simulink model "ddc_bpm_476_066"  (Simulink 7.8)
settings: Solver=ode45  StartTime=0.0  StopTime=2e-3  RelTol=1e-3
undefined symbols (not defined in the file): decim_factor_poly_35, dt_sim, frev_476, Fs_adc, n_ch, n_ovs, R_fofb, R_sec, R_sec_cfir, R_sec_pfir, xlipgetpartsetting
libraries: xbsIndex_r4 x1436, simulink x7
(part 12 of 12)

== system ddc_bpm_476_066/TBT_amp/TBT_amp1/TBT_poly_decim/TDDM_TBT/TDDM_tbt_poly_i ==
  din : Inport
  ch_in : Inport  Port=2
  Constant : xbsIndex_r4/Constant  const=1  gui_display_data_type=Fixed-point  arith_type=Unsigned  n_bits=1  bin_pt=0  preci_type=Single  exp_width=8  frac_width=24  explicit_period=off  period=1  equ=P=C  opselect=C  inp2=PCIN>>17  opr=+  inp1=P  carry=CIN  dbl_ovrd=off  block_type=constant
  Constant1 : xbsIndex_r4/Constant  const=0  gui_display_data_type=Fixed-point  arith_type=Unsigned  n_bits=1  bin_pt=0  preci_type=Single  exp_width=8  frac_width=24  explicit_period=off  period=1  equ=P=C  opselect=C  inp2=PCIN>>17  opr=+  inp1=P  carry=CIN  dbl_ovrd=off  block_type=constant
  Delay : xbsIndex_r4/Delay  rst=off  infoeditControl=Selection of Reset will increase slice count due to use of real FFs and instead of SRLs  en=off  latency=3  dbl_ovrd=off  reg_retiming=off  block_type=delay
  Down Sample1 : xbsIndex_r4/Down Sample  sample_ratio=n_ch/n_ovs  sample_phase="Last Value of Frame  (most efficient)"  en=off  latency=1  dbl_ovrd=off  block_type=dsamp
  Down Sample2 : xbsIndex_r4/Down Sample  sample_ratio=n_ch/n_ovs  sample_phase="Last Value of Frame  (most efficient)"  en=off  latency=1  dbl_ovrd=off  block_type=dsamp
  Register : xbsIndex_r4/Register  init=0  rst=off  en=on  dbl_ovrd=off  block_type=register
  Register1 : xbsIndex_r4/Register  init=0  rst=off  en=on  dbl_ovrd=off  block_type=register
  Relational : xbsIndex_r4/Relational  mode=a=b  en=off  latency=1  dbl_ovrd=off  block_type=relational
  Relational1 : xbsIndex_r4/Relational  mode=a=b  en=off  latency=1  dbl_ovrd=off  block_type=relational
  dout_ch0 : Outport
  dout_ch1 : Outport  Port=2
  ch_out : Outport  Port=3
  wires:
  Constant/1 -> Relational/2
  Constant1/1 -> Relational1/2
  Relational/1 -> Register/2
  Relational1/1 -> Register1/2
  din/1 -> Register/1, Register1/1
  Register/1 -> Down Sample2/1
  ch_in/1 -> Relational/1, Relational1/1, Delay/1
  Register1/1 -> Down Sample1/1
  Down Sample2/1 -> dout_ch0/1
  Delay/1 -> ch_out/1
  Down Sample1/1 -> dout_ch1/1

== system ddc_bpm_476_066/TBT_amp/TBT_amp1/TBT_poly_decim/TDDM_TBT/TDDM_tbt_poly_q ==
  din : Inport
  ch_in : Inport  Port=2
  Constant : xbsIndex_r4/Constant  const=1  gui_display_data_type=Fixed-point  arith_type=Unsigned  n_bits=1  bin_pt=0  preci_type=Single  exp_width=8  frac_width=24  explicit_period=off  period=1  equ=P=C  opselect=C  inp2=PCIN>>17  opr=+  inp1=P  carry=CIN  dbl_ovrd=off  block_type=constant
  Constant1 : xbsIndex_r4/Constant  const=0  gui_display_data_type=Fixed-point  arith_type=Unsigned  n_bits=1  bin_pt=0  preci_type=Single  exp_width=8  frac_width=24  explicit_period=off  period=1  equ=P=C  opselect=C  inp2=PCIN>>17  opr=+  inp1=P  carry=CIN  dbl_ovrd=off  block_type=constant
  Delay : xbsIndex_r4/Delay  rst=off  infoeditControl=Selection of Reset will increase slice count due to use of real FFs and instead of SRLs  en=off  latency=3  dbl_ovrd=off  reg_retiming=off  block_type=delay
  Down Sample1 : xbsIndex_r4/Down Sample  sample_ratio=n_ch/n_ovs  sample_phase="Last Value of Frame  (most efficient)"  en=off  latency=1  dbl_ovrd=off  block_type=dsamp
  Down Sample2 : xbsIndex_r4/Down Sample  sample_ratio=n_ch/n_ovs  sample_phase="Last Value of Frame  (most efficient)"  en=off  latency=1  dbl_ovrd=off  block_type=dsamp
  Register : xbsIndex_r4/Register  init=0  rst=off  en=on  dbl_ovrd=off  block_type=register
  Register1 : xbsIndex_r4/Register  init=0  rst=off  en=on  dbl_ovrd=off  block_type=register
  Relational : xbsIndex_r4/Relational  mode=a=b  en=off  latency=1  dbl_ovrd=off  block_type=relational
  Relational1 : xbsIndex_r4/Relational  mode=a=b  en=off  latency=1  dbl_ovrd=off  block_type=relational
  dout_ch0 : Outport
  dout_ch1 : Outport  Port=2
  ch_out : Outport  Port=3
  wires:
  Constant/1 -> Relational/2
  Constant1/1 -> Relational1/2
  Relational/1 -> Register/2
  Relational1/1 -> Register1/2
  din/1 -> Register/1, Register1/1
  Register/1 -> Down Sample2/1
  ch_in/1 -> Relational/1, Relational1/1, Delay/1
  Register1/1 -> Down Sample1/1
  Down Sample2/1 -> dout_ch0/1
  Delay/1 -> ch_out/1
  Down Sample1/1 -> dout_ch1/1
